simulink model "test"  (R2023b)
settings: Solver=ode4  StartTime=0.0  StopTime=1  FixedStep=0.1  RelTol=1e-3
settings Model: Creator=HP  LastModifiedBy=HP

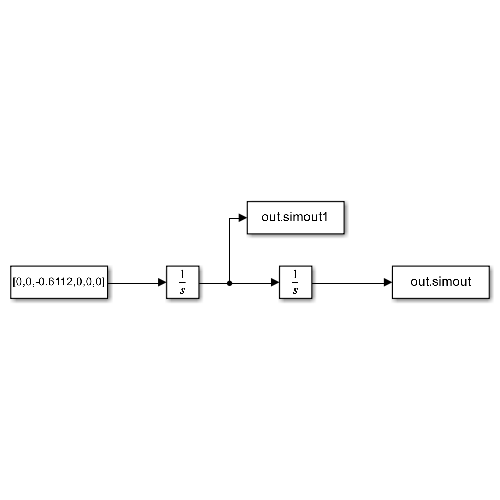
[thumbnail: Simulink's stored preview of the top-level diagram]
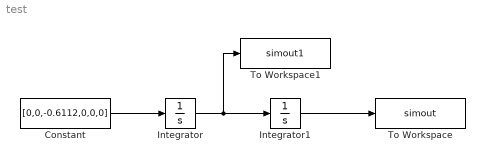
== system test ==
  Constant : Constant  Value=[0,0,-0.6112,0,0,0]
  Integrator : Integrator  InitialCondition=[0,0,0,0,0,0]
  Integrator1 : Integrator  InitialCondition=[0,0,0,0,0,0]
  To Workspace : ToWorkspace  VariableName=simout  SampleTime=-1
  To Workspace1 : ToWorkspace  VariableName=simout1  SampleTime=-1
  wires:
  Constant/1 -> Integrator/1
  Integrator/1 -> To Workspace1/1, Integrator1/1
  Integrator1/1 -> To Workspace/1
